simulink library "mech_stewart_control_equil_leg"  (Simulink 6.0)
settings: Solver=ode45  SolverMode=SingleTasking  StartTime=0.0  StopTime=10.0  RelTol=1e-3
values from neighbouring files (symbols this model uses):
  m = 161    [mech_transmission_data.mat]
  N = 270    [mech_transmission_data.mat]
undefined symbols (not defined in the file or in its folder): lower_leg_inertia, lower_leg_mass, upper_leg_inertia, upper_leg_mass
libraries: mblibv1 x7
settings Model: Creator=jwendlan  LastModifiedBy=batserve  ExtModeAutoUpdateStatusClock=off
settings OptimizationCC: BooleanDataType=off
settings DebuggingCC: SolverPrmCheckMsg=none
settings HardwareCC: TargetUnknown=on

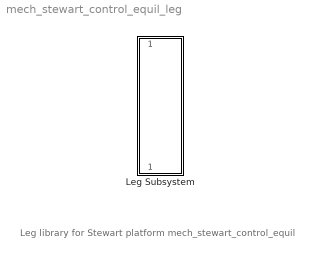
== system mech_stewart_control_equil_leg ==
  note: Leg library for Stewart platform
      | mech_stewart_control_equil
  Leg Subsystem : Subsystem  Orientation=down  mask{ln=1}
      mask prompts: ln "Leg Number"

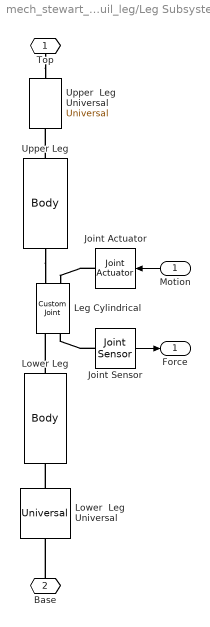
== system mech_stewart_control_equil_leg/Leg Subsystem ==
  Motion : Inport  Description=Applies a force (N) to the prismatic axis  Orientation=left  Port=1  LatchInput=off
  Joint Actuator : mblibv1/Sensors &  Actuators/Joint Actuator  Orientation=left  Opaque=on  PortType=blob  PhysicalDomain=Mechanical  ActuationStyle=Motion  AngleUnits=deg  ArcVelocityUnits=deg/s  ArcAccelerationUnits=deg/s^2  CoordPositionUnits=m  VelocityUnits=m/s  AccelerationUnits=m/s^2  ForceUnits=N  TorqueUnits=N-m  ActiveIO=off  Width=1  DialogClass=MechanicalActuatorBlock  Primitive=P1  ReferenceFrame=Absolute (INERTIAL)
  Joint Sensor : mblibv1/Sensors &  Actuators/Joint Sensor  Opaque=on  PortType=blob  PhysicalDomain=Mechanical  Muxed=on  Pose=off  Angle=on  AngleUnits=deg  ArcVelocity=off  ArcVelocityUnits=deg/s  ArcAcceleration=off  ArcAccelerationUnits=deg/s^2  CoordPosition=off  CoordPositionUnits=m  Velocity=off  VelocityUnits=m/s  Acceleration=off  AccelerationUnits=m/s^2  Quaternion=on  QuaternionDT=off  QuaternionDDT=off  QuaternionUnits=off  OutputVector=[ 1 ]  ActiveIO=off  Width=1  DialogClass=MechanicalSensorBlock  Primitive=P1  Force=on  ForceUnits=N  Torque=off  TorqueUnits=N-m  ReferenceFrame=Absolute (INERTIAL)  ReactionSensedSide=Base  ReactionReferenceFrame=Absolute (World)  ReactionForce=off  ReactionForceUnits=N  ReactionMoment=off  ReactionMomentUnits=N-m
  Leg Cylindrical : mblibv1/Joints/Custom Joint  Orientation=up  PhysicalDomain=mechanical  SubClassName=custom_joint  LeftPortType=blob  RightPortType=blob  LConnTagsString=__newl0|SA1  RConnTagsString=__newr0|SA1  NumSAPorts=2  CutJoint=off  MarkAsCut=off  Primitives=revolute_prismatic  PrimitiveProps=R1$WORLD$cyl1(ln,:)$revolute#P1$WORLD$cyl1(ln,:)$prismatic  DialogClass=JointBlock
  Lower Leg : mblibv1/Bodies/Body  Orientation=up  PhysicalDomain=mechanical  SubClassName=Unknown  LeftPortType=workingframe  RightPortType=workingframe  LConnTagsString=CS1  RConnTagsString=CS3  DialogClass=MechanicalBodyBlock  Mass=lower_leg_mass  MassUnits=kg  InertiaUnits=kg*m^2  Inertia=lower_leg_inertia  Shape=Cylinder  ShapeDims=[1 1]  ShapeUnits=m  ShapeUse=false  Density=1  DensityUnits=kg/m^3  DensityUse=false  CG=Left$CG$lower_leg(ln).origin$WORLD$WORLD$m$lower_leg(ln).rotation$3x3 Transform$deg$WORLD$false  WorkingFrames=Left$CS1$pos_base(ln,:)$WORLD$WORLD$m$lower_leg(ln).rotation$3x3 Transform$deg$WORLD$true#Right$CS3$(lower_leg(ln).end_point + upper_leg(ln).end_point)/2$WORLD$WORLD$m$lower_leg(ln).rotation$3x3 Transform$deg$WORLD$true#Right$CS2$lower_leg(ln).end_point$WORLD$WORLD$m$lower_leg(ln).rotation$3x3 Transform$deg$WORLD$false
  Lower  Leg Universal : mblibv1/Joints/Universal  Orientation=up  PhysicalDomain=mechanical  SubClassName=Unknown  LeftPortType=blob  RightPortType=blob  LConnTagsString=__newl0  RConnTagsString=__newr0  NumSAPorts=0  CutJoint=off  MarkAsCut=off  Primitives=revolute_revolute  PrimitiveProps=R1$WORLD$rev1(ln,:)$revolute#R2$WORLD$rev2(ln,:)$revolute  DialogClass=JointBlock
  Upper Leg : mblibv1/Bodies/Body  Orientation=up  PhysicalDomain=mechanical  SubClassName=Unknown  LeftPortType=workingframe  RightPortType=workingframe  LConnTagsString=CS3  RConnTagsString=CS2  DialogClass=MechanicalBodyBlock  Mass=upper_leg_mass  MassUnits=kg  InertiaUnits=kg*m^2  Inertia=upper_leg_inertia  Shape=Cylinder  ShapeDims=[1 1]  ShapeUnits=m  ShapeUse=false  Density=1  DensityUnits=kg/m^3  DensityUse=false  CG=Left$CG$upper_leg(ln).origin$WORLD$WORLD$m$upper_leg(ln).rotation$3x3 Transform$deg$WORLD$false  WorkingFrames=Left$CS3$(lower_leg(ln).end_point + upper_leg(ln).end_point)/2$WORLD$WORLD$m$upper_leg(ln).rotation$3x3 Transform$deg$WORLD$true#Left$CS1$upper_leg(ln).end_point$WORLD$WORLD$m$upper_leg(ln).rotation$3x3 Transform$deg$WORLD$false#Right$CS2$pos_top(ln,:)$WORLD$WORLD$m$upper_leg(ln).rotation$3x3 Transform$deg$WORLD$true
  Upper  Leg Universal : mblibv1/Joints/Universal  Orientation=up  PhysicalDomain=mechanical  SubClassName=Unknown  LeftPortType=blob  RightPortType=blob  LConnTagsString=__newl0  RConnTagsString=__newr0  NumSAPorts=0  CutJoint=off  MarkAsCut=off  Primitives=revolute_revolute  PrimitiveProps=R1$WORLD$rev3(ln,:)$revolute#R2$WORLD$rev4(ln,:)$revolute  DialogClass=JointBlock
  Top : PMIOPort  Orientation=down  Port=1  Side=Left
  Base : PMIOPort  Orientation=up  Port=2  Side=Right
  Force : Outport  Description=Senses position and velocity of the prismatic axis
  wires:
  Motion/1 -> Joint Actuator/1
  Joint Sensor/1 -> Force/1
  connections:
  Lower  Leg Universal/RConn1 -- Lower Leg/LConn1
  Upper Leg/RConn1 -- Upper  Leg Universal/LConn1
  Top/RConn1 -- Upper  Leg Universal/RConn1
  Base/RConn1 -- Lower  Leg Universal/LConn1
  Joint Actuator/RConn1 -- Leg Cylindrical/RConn2
  Joint Sensor/LConn1 -- Leg Cylindrical/LConn2
  Lower Leg/RConn1 -- Leg Cylindrical/LConn1
  Upper Leg/LConn1 -- Leg Cylindrical/RConn1
